simulink model "task2"  (R2024a)
settings: Solver=VariableStepAuto  StartTime=0.0  StopTime=10  RelTol=1e-6
values from neighbouring files (symbols this model uses):
  A = [-40, 16, 9, 7; -64, 25, 14 ,12; -26, 11, 7, 3; -48, 18, 14, 8]    [main.m]
  C = [-3, 2, -2, 1]    [main.m]
  L = L3    [main.m]
settings Model: Creator=alexivanov  LastModifiedBy=alexivanov

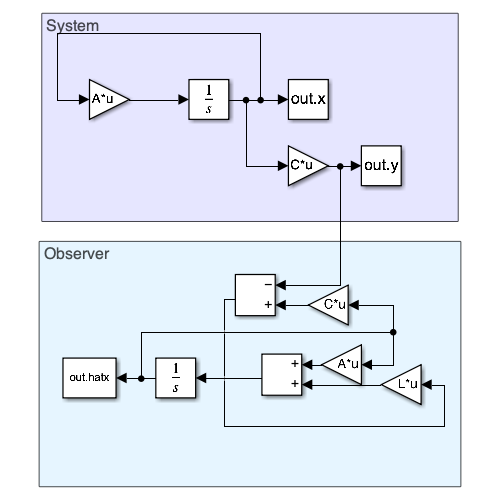
[thumbnail: Simulink's stored preview of the top-level diagram]
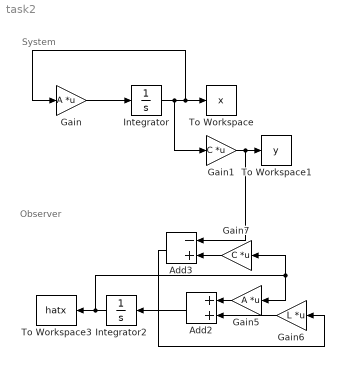
== system task2 ==
  note: Observer
  note: System
  Add2 : Sum
  Add3 : Sum  Inputs=-+
  Gain : Gain  Gain=A  Multiplication=Matrix(K*u)
  Gain1 : Gain  Gain=C  Multiplication=Matrix(K*u)
  Gain5 : Gain  Gain=A  Multiplication=Matrix(K*u)
  Gain6 : Gain  Gain=L  Multiplication=Matrix(K*u)
  Gain7 : Gain  Gain=C  Multiplication=Matrix(K*u)
  Integrator : Integrator  InitialCondition=[1; 1; 1; 1]
  Integrator2 : Integrator  InitialCondition=[2; 0; 0; -1]
  To Workspace : ToWorkspace  VariableName=x  SampleTime=-1
  To Workspace1 : ToWorkspace  VariableName=y  SampleTime=-1
  To Workspace3 : ToWorkspace  VariableName=hatx  SampleTime=-1
  wires:
  Gain/1 -> Integrator/1
  Gain1/1 -> Add3/1, To Workspace1/1
  Integrator/1 -> Gain1/1, Gain/1, To Workspace/1
  Gain5/1 -> Add2/1
  Gain6/1 -> Add2/2
  Add2/1 -> Integrator2/1
  Gain7/1 -> Add3/2
  Add3/1 -> Gain6/1
  Integrator2/1 -> Gain5/1, Gain7/1, To Workspace3/1
